simulink model "mass_spring6"  (R2022b)
settings: Solver=VariableStepAuto  StartTime=0.0  StopTime=Sim_Tim  RelTol=1e-3
undefined symbols (not defined in the file): b1, b2, F, k1, k2, m1, m2
settings Model: Creator=HashimAbdulAzizHashi  LastModifiedBy=HashimAbdulAzizHashi

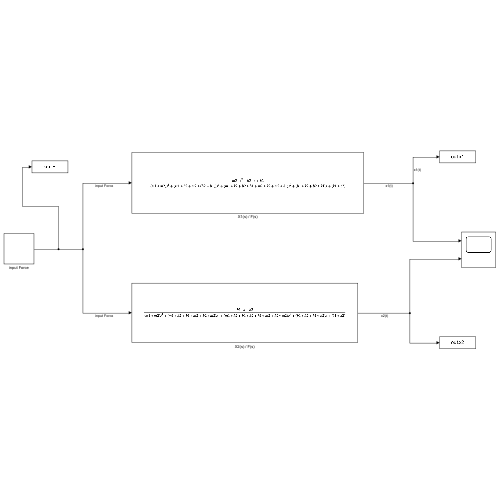
[thumbnail: Simulink's stored preview of the top-level diagram]
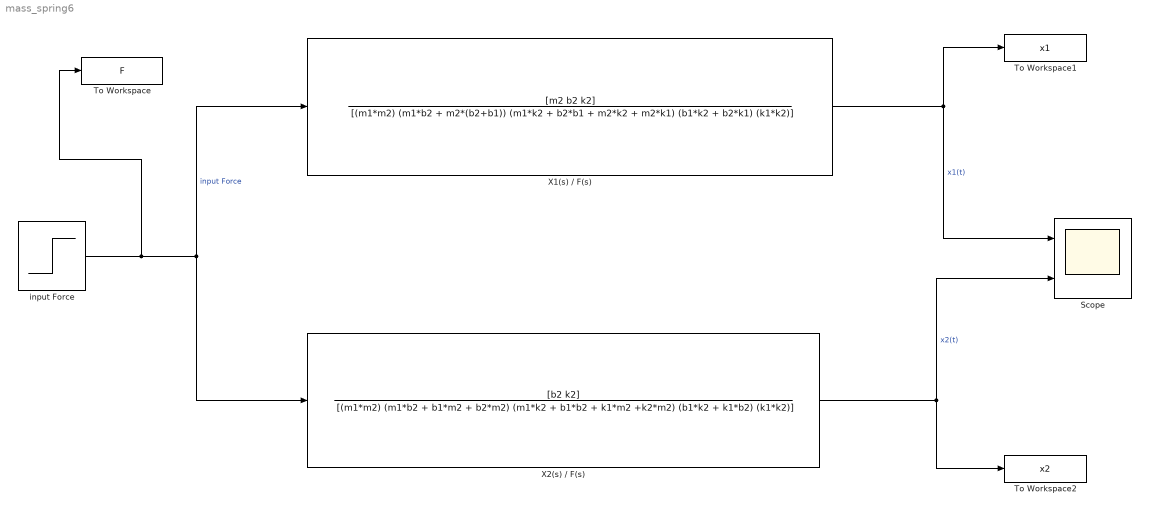
== system mass_spring6 ==
  Scope : Scope  NumInputPorts=2
  To Workspace : ToWorkspace  VariableName=F  SaveFormat=Timeseries  SampleTime=-1
  To Workspace1 : ToWorkspace  VariableName=x1  SaveFormat=Timeseries  SampleTime=-1
  To Workspace2 : ToWorkspace  VariableName=x2  SaveFormat=Timeseries  SampleTime=-1
  X1(s) / F(s) : TransferFcn  Numerator=[m2 b2 k2]  Denominator=[(m1*m2) (m1*b2 + m2*(b2+b1)) (m1*k2 + b2*b1 + m2*k2 + m2*k1) (b1*k2 + b2*k1) (k1*k2)]
  X2(s) / F(s) : TransferFcn  Numerator=[b2 k2]  Denominator=[(m1*m2) (m1*b2 + b1*m2 + b2*m2) (m1*k2 + b1*b2 + k1*m2 +k2*m2) (b1*k2 + k1*b2) (k1*k2)]
  input Force : Step  After=F  SampleTime=0
  wires:
  input Force/1 -> To Workspace/1, X2(s) / F(s)/1, X1(s) / F(s)/1  "input Force"
  X1(s) / F(s)/1 -> To Workspace1/1, Scope/1  "x1(t)"
  X2(s) / F(s)/1 -> To Workspace2/1, Scope/2  "x2(t)"
